simulink model "Zad_6_sch"  (R2022a)
settings: Solver=VariableStepAuto  StartTime=0.0  StopTime=10.0  MaxStep=0.001  RelTol=1e-3
values from neighbouring files (symbols this model uses):
  a21 = (1/(2*m))*x30^2*(FemP1/FemP2^2)*exp(-x10/FemP2)    [Zad_2.m]
  a23 = -(1/m)*x30*(FemP1/FemP2)*exp(-x10/FemP2)    [Zad_2.m]
  a31 = (1/f1)*exp(x10/f2)*(ki*u10+ci-x30)    [Zad_2.m]
  a33 = -(f2/f1)*exp(x10/f2)    [Zad_2.m]
  b31 = ki*(f2/f1)*exp(x10/f2)    [Zad_2.m]
  g = 9.81    [Zad_2.m]
  K1 = 1    [Zad_4.m]
  K3g = -1/a23    [Zad_4.m]
  K3yr = -a21/a23    [Zad_4.m]
  Kg = a33/(a23*b31)    [Zad_4.m]
  Kxpom = place(A,Bpom,p_d)    [Zad_4.m]    (also in Zad_5.m; Zad_6.m)
  Kyr = (a21*a33-a31*a23)/(a23*b31)    [Zad_4.m]
  Tp = 0.0001    [Zad_5.m]    (also in Zad_6.m = 0.001)
  xd = d-bd    (= 0.01326)    [Zad_2.m]
settings Model: Creator=marci  LastModifiedBy=marci

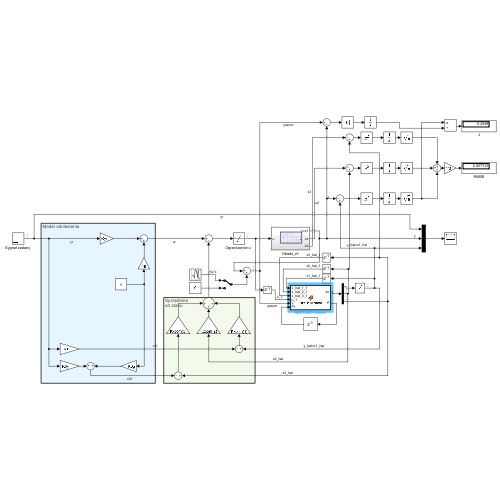
[thumbnail: Simulink's stored preview of the top-level diagram]
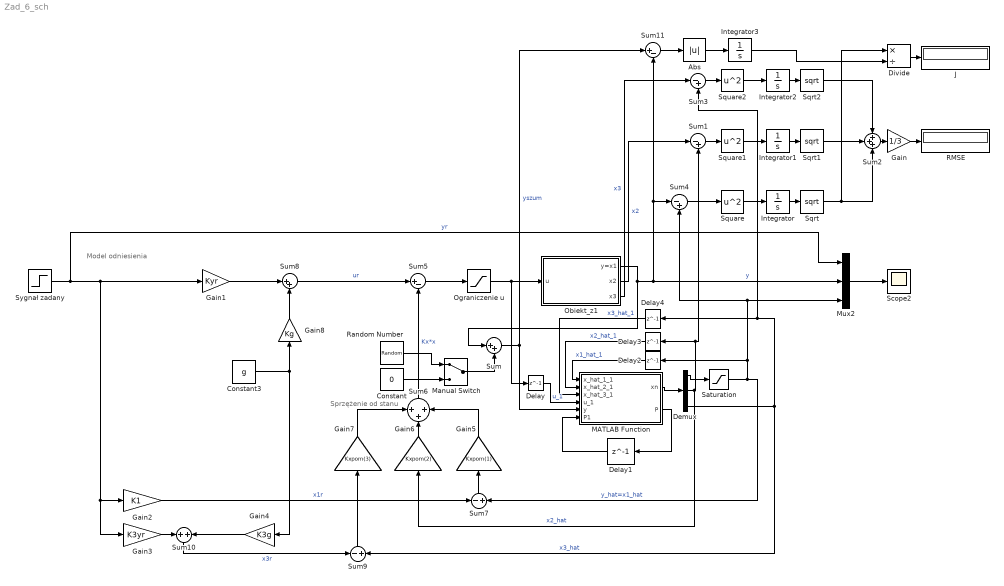
== system Zad_6_sch ==
  note: Sprzężenie
      | od stanu
  note: Model odniesienia
  " Sygnał zadany  " : Step  Time=0  After=0.008  SampleTime=0
  Abs : Abs  SaturateOnIntegerOverflow=off
  Constant : Constant  Value=0
  Constant3 : Constant  Value=g
  Delay : Delay  DelayLength=1  SampleTime=Tp
  Delay1 : Delay  DelayLength=1  InitialCondition=[0.0 0.0 0.0; 0.0 0.0 0.0; 0.0 0.0 0.0]  SampleTime=Tp
  Delay2 : Delay  DelayLength=1  InitialCondition=xd  SampleTime=Tp
  Delay3 : Delay  DelayLength=1  SampleTime=Tp
  Delay4 : Delay  DelayLength=1  SampleTime=Tp
  Demux : Demux  Outputs=3
  Divide : Product  Inputs=*/
  Gain : Gain  Gain=1/3
  Gain1 : Gain  Gain=Kyr
  Gain2 : Gain  Gain=K1
  Gain3 : Gain  Gain=K3yr
  Gain4 : Gain  Gain=K3g
  Gain5 : Gain  Gain=Kxpom(1)
  Gain6 : Gain  Gain=Kxpom(2)
  Gain7 : Gain  Gain=Kxpom(3)
  Gain8 : Gain  Gain=Kg
  Integrator{,1..3} (4 alike) : Integrator
  J : Display
  MATLAB Function : MATLAB Function  TreatAsAtomicUnit=on  SystemSampleTime=0.0001
  Manual Switch : ManualSwitch
  Mux2 : Mux  Inputs=3
  Obiekt_z1 : Subsystem
  "Ograniczenie u  " : Saturate  UpperLimit=1  LowerLimit=0  ZeroCross=off
  RMSE : Display
  Random Number : RandomNumber  Variance=1e-8  SampleTime=0.001
  Saturation : Saturate  UpperLimit=xd  LowerLimit=0
  Scope2 : Scope
  Sqrt : Sqrt
  Sqrt1 : Sqrt
  Sqrt2 : Sqrt
  Square : Math  Operator=square
  Square1 : Math  Operator=square
  Square2 : Math  Operator=square
  Sum : Sum  Inputs=|++
  Sum1 : Sum  Inputs=|-+
  Sum10 : Sum
  Sum11 : Sum  Inputs=|+-
  Sum2 : Sum  Inputs=+++
  Sum3 : Sum  Inputs=|-+
  Sum4 : Sum  Inputs=|-+
  Sum5 : Sum  Inputs=|+-
  Sum6 : Sum  Inputs=+++
  Sum7 : Sum  Inputs=-+
  Sum8 : Sum  Inputs=|++
  Sum9 : Sum  Inputs=-+
  wires:
  Sum8/1 -> Sum5/1  "ur"
  "Ograniczenie u  "/1 -> Delay/1, Obiekt_z1/1(u)
  Demux/1 -> Saturation/1
  Demux/2 -> Gain6/1, Delay3/1, Sum1/2  "x2_hat"
  Gain7/1 -> Sum6/1
  Demux/3 -> Sum3/2, Delay4/1, Sum9/2  "x3_hat"
  Gain3/1 -> Sum10/1
  Gain8/1 -> Sum8/2
  Gain5/1 -> Sum6/3
  Delay2/1 -> MATLAB Function/1(x_hat_1_1)  "x1_hat_1"
  Delay3/1 -> MATLAB Function/2(x_hat_2_1)  "x2_hat_1"
  Obiekt_z1/1(y=x1) -> Sum11/2, Sum4/1, Mux2/2, Sum/1  "y"
  MATLAB Function/1(xn) -> Demux/1
  Gain1/1 -> Sum8/1
  Mux2/1 -> Scope2/1
  Sum6/1 -> Sum5/2  "Kx*x"
  Sum5/1 -> "Ograniczenie u  "/1
  Gain6/1 -> Sum6/2
  Sum4/1 -> Square/1
  Sum10/1 -> Sum9/1  "x3r"
  Sum9/1 -> Gain7/1
  Gain4/1 -> Sum10/2
  Sum7/1 -> Gain5/1
  Constant3/1 -> Gain4/1, Gain8/1
  " Sygnał zadany  "/1 -> Mux2/1, Gain1/1, Gain3/1, Gain2/1  "yr"
  Saturation/1 -> Sum7/2, Mux2/3, Sum4/2, Delay2/1  "y_hat=x1_hat"
  Delay/1 -> MATLAB Function/4(u_1)  "u_1"
  Delay4/1 -> MATLAB Function/3(x_hat_3_1)  "x3_hat_1"
  Gain2/1 -> Sum7/1  "x1r"
  MATLAB Function/2(P) -> Delay1/1
  Delay1/1 -> MATLAB Function/6(P1)
  Sum/1 -> Sum11/1, MATLAB Function/5(y)  "yszum"
  Manual Switch/1 -> Sum/2
  Constant/1 -> Manual Switch/2
  Random Number/1 -> Manual Switch/1
  Square/1 -> Integrator/1
  Integrator/1 -> Sqrt/1
  Sqrt/1 -> Sum2/3, Divide/1
  Obiekt_z1/2(x2) -> Sum1/1  "x2"
  Integrator1/1 -> Sqrt1/1
  Square1/1 -> Integrator1/1
  Sum1/1 -> Square1/1
  Sum2/1 -> Gain/1
  Gain/1 -> RMSE/1
  Sqrt1/1 -> Sum2/2
  Integrator2/1 -> Sqrt2/1
  Square2/1 -> Integrator2/1
  Sum3/1 -> Square2/1
  Sqrt2/1 -> Sum2/1
  Obiekt_z1/3(x3) -> Sum3/1  "x3"
  Sum11/1 -> Abs/1
  Abs/1 -> Integrator3/1
  Integrator3/1 -> Divide/2
  Divide/1 -> J/1

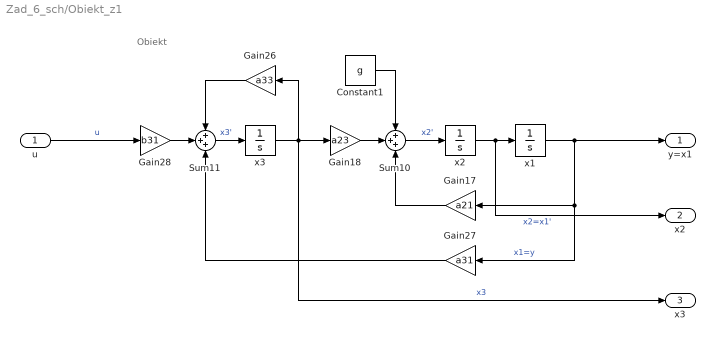
== system Zad_6_sch/Obiekt_z1 ==
  note: Obiekt
  u : Inport
  " x1" : Integrator  InitialCondition=xd  LimitOutput=on  UpperSaturationLimit=xd  LowerSaturationLimit=0
  " x2" : Integrator
  " x3" : Integrator
  Constant1 : Constant  Value=g
  Gain17 : Gain  Gain=a21
  Gain18 : Gain  Gain=a23
  Gain26 : Gain  Gain=a33
  Gain27 : Gain  Gain=a31
  Gain28 : Gain  Gain=b31
  Sum10 : Sum  Inputs=+++
  Sum11 : Sum  Inputs=+++
  y=x1 : Outport
  x2 : Outport  Port=2
  x3 : Outport  Port=3
  wires:
  Gain18/1 -> Sum10/2
  " x2"/1 -> x2/1, " x1"/1  "x2=x1'"
  u/1 -> Gain28/1  "u"
  " x1"/1 -> y=x1/1, Gain17/1, Gain27/1  "x1=y"
  Sum10/1 -> " x2"/1  "x2'"
  Gain28/1 -> Sum11/2
  Gain17/1 -> Sum10/3
  " x3"/1 -> x3/1, Gain18/1, Gain26/1  "x3"
  Constant1/1 -> Sum10/1
  Gain26/1 -> Sum11/1
  Gain27/1 -> Sum11/3
  Sum11/1 -> " x3"/1  "x3'"

== matlab function Zad_6_sch/MATLAB Function ==
  data: x_hat_1_1 input; xn output; x_hat_2_1 input; x_hat_3_1 input; u_1 input; y input; P1 input; P output
function [xn,P]=Filtr_Kalmana(x_hat_1_1, x_hat_2_1, x_hat_3_1, u_1, y,P1)
%funkcja bedaca filtrem Kalmana

%Macierze modelu ciaglego
A=[0,1,0;3.198854799795517e+03,0,-49.672670359171390;0,0,-1.862601595234874e+02];
B=[0,0;0,9.810000000000000;4.687236914408560e+02,0];
C=[1,0,0];

%Dyskretyzacja modelu
Tp=0.001; %okres probkowania
Ad=eye(3)+A*Tp;
Bd=B*Tp;
Cd=C;

u_pom=[u_1; 1];
x_hat1=[x_hat_1_1; x_hat_2_1; x_hat_3_1];

%Tutaj mozna dobrac macierze Q i R
Q=diag([0.000001 0.000001 0.000001]); %macierz kowariancji szumów przetwarzania
R=0.01; %macierz kowariancji szumów pomiarowych

%Etap predykcji
x_pom=Ad*x_hat1+Bd*u_pom;
P_pom=Ad*P1*Ad'+Q;

%Etap filtracji
K=P_pom*Cd'*(Cd*P_pom*Cd'+R)^(-1);
xn=x_pom+K*(y-Cd*x_pom);
P=(eye(3)-K*Cd)*P_pom;
end
